simulink model "curr_vel_pos_cascaded"  (R2023b)
settings: Solver=VariableStepAuto  StartTime=0.0  StopTime=10  FixedStep=0.00001  RelTol=0.001
undefined symbols (not defined in the file or in its folder): d_theta, dd_theta, Fm, Im, theta
libraries: cstblocks x14
settings Model: Creator=frenci  LastModifiedBy=frenc

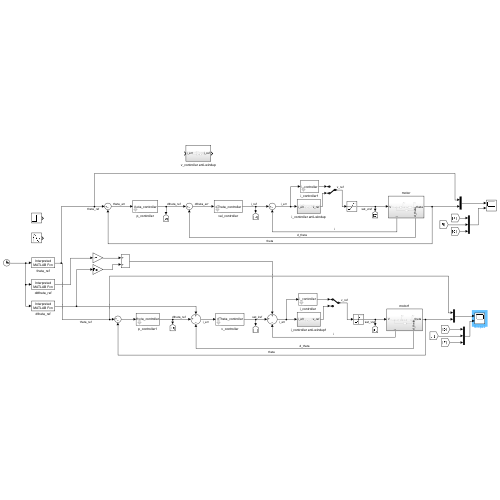
[thumbnail: Simulink's stored preview of the top-level diagram]
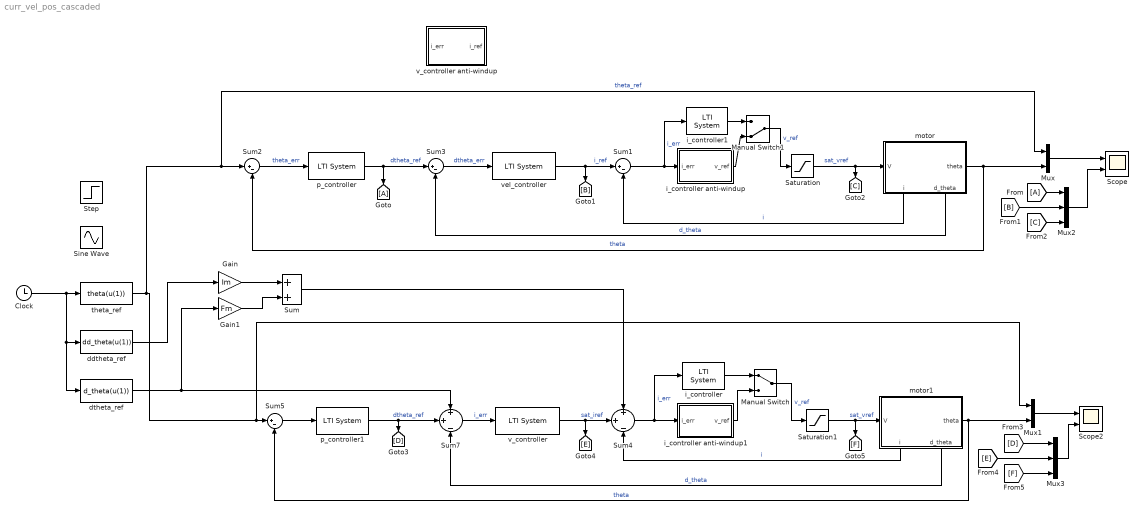
== system curr_vel_pos_cascaded ==
  Clock : Clock
  From : From
  Gain : Gain  Gain=Im
  Gain1 : Gain  Gain=Fm
  Goto : Goto
  Manual Switch : ManualSwitch
  Manual Switch1 : ManualSwitch  CurrentSetting=0
  Mux : Mux  Inputs=2
  Mux1 : Mux  Inputs=2
  Mux2 : Mux  Inputs=3
  Mux3 : Mux  Inputs=3
  Saturation : Saturate  UpperLimit=20  LowerLimit=-20
  Saturation1 : Saturate  UpperLimit=20  LowerLimit=-20
  Scope : Scope  NumInputPorts=2
  Scope2 : Scope  NumInputPorts=2
  Sine Wave : Sin  Amplitude=0.02  Frequency=2*pi*10  SampleTime=0
  Step : Step  Time=0.01  SampleTime=0
  Sum : Sum  Inputs=|+|+|
  Sum{1..3,5} (4 alike) : Sum  Inputs=|+-
  Sum4 : Sum  Inputs=+|+|-
  Sum7 : Sum  Inputs=+|+|-
  ddtheta_ref : MATLABFcn  MATLABFcn=dd_theta(u(1))
  dtheta_ref : MATLABFcn  MATLABFcn=d_theta(u(1))
  i_controller : cstblocks/LTI System  sys=i_controller  IC=[]  PadeOrder=0
  i_controller anti-windup : Subsystem
  i_controller anti-windup1 : Subsystem
  i_controller1 : cstblocks/LTI System  sys=i_controller  IC=[]  PadeOrder=0
  motor : Subsystem
      settings: PortSchema="{\"entries\":[{\"content\":{\"sides\":[{\"content\":{\"connectorIds\":[\"In1\"]},\"type\":\"ConnectorPlacement.EquallySpacedRectSide\",\"uuid\":\"f8a2075c-835e-4141-b12e-4d20e284e554\"},{\"content\":{\"connectorIds\":[\"Out1\"],\"side\":\"RIGHT\"},\"type\":\"ConnectorPlacement.EquallySpacedRectSide\",\"uuid\":\"7d0ccdb0-5eec-43bf-a9a0-3828bb795771\"},{\"content\":{\"side\":\"TOP\"},\"type\":\"ConnectorPlacement.EquallySpacedRectSide\",\"uuid\":\"6f2e9e0d-bcbc-45fe-ae47-d363e6343883\"},{\"content\":{\"connectorIds\":[\"Out2\",\"Out3\"],\"side\":\"BOTTOM\"},\"type\":\"ConnectorPlacement.EquallySpacedRectSide\",\"uuid\":\"12f63cf8-6157-4e53-9068-17bec2e9afdd\"}]},\"type\":\"ConnectorPlacement.EquallySpacedConnector\",\"uuid\":\"d79290fb-8e13-45e0-9c36-c4b7a16caadb\"}],\"packageUris\":[\"http://schema.mathworks.com/mf0/Connector/R2020b\"],\"version\":\"1.0\"}"
  motor1 : Subsystem
      settings: PortSchema="{\"entries\":[{\"content\":{\"sides\":[{\"content\":{\"connectorIds\":[\"In1\"]},\"type\":\"ConnectorPlacement.EquallySpacedRectSide\",\"uuid\":\"f8a2075c-835e-4141-b12e-4d20e284e554\"},{\"content\":{\"connectorIds\":[\"Out1\"],\"side\":\"RIGHT\"},\"type\":\"ConnectorPlacement.EquallySpacedRectSide\",\"uuid\":\"7d0ccdb0-5eec-43bf-a9a0-3828bb795771\"},{\"content\":{\"side\":\"TOP\"},\"type\":\"ConnectorPlacement.EquallySpacedRectSide\",\"uuid\":\"6f2e9e0d-bcbc-45fe-ae47-d363e6343883\"},{\"content\":{\"connectorIds\":[\"Out2\",\"Out3\"],\"side\":\"BOTTOM\"},\"type\":\"ConnectorPlacement.EquallySpacedRectSide\",\"uuid\":\"12f63cf8-6157-4e53-9068-17bec2e9afdd\"}]},\"type\":\"ConnectorPlacement.EquallySpacedConnector\",\"uuid\":\"d79290fb-8e13-45e0-9c36-c4b7a16caadb\"}],\"packageUris\":[\"http://schema.mathworks.com/mf0/Connector/R2020b\"],\"version\":\"1.0\"}"
  p_controller : cstblocks/LTI System  sys=theta_controller  IC=[]  PadeOrder=0
  p_controller1 : cstblocks/LTI System  sys=theta_controller  IC=[]  PadeOrder=0
  theta_ref : MATLABFcn  MATLABFcn=theta(u(1))
  v_controller : cstblocks/LTI System  sys=dTheta_controller  IC=[]  PadeOrder=0
  v_controller anti-windup : Subsystem
  vel_controller : cstblocks/LTI System  sys=dTheta_controller  IC=[]  PadeOrder=0
  wires:
  Sum2/1 -> p_controller/1  "theta_err"
  Mux/1 -> Scope/1
  motor/2(i) -> Sum1/2  "i"
  Saturation/1 -> [C], motor/1(V)  "sat_vref"
  vel_controller/1 -> Sum1/1, [B]  "i_ref"
  Sum1/1 -> i_controller1/1, i_controller anti-windup/1(i_err)  "i_err"
  i_controller anti-windup/1(v_ref) -> Manual Switch1/2
  Sum3/1 -> vel_controller/1  "dtheta_err"
  motor1/1(theta) -> Mux1/2, Sum5/2  "theta"
  Sum5/1 -> p_controller1/1
  motor1/2(i) -> Sum4/3  "i"
  Mux1/1 -> Scope2/1
  Saturation1/1 -> [F], motor1/1(V)  "sat_vref"
  p_controller1/1 -> Sum7/2, [D]  "dtheta_ref"
  v_controller/1 -> Sum4/2, [E]  "sat_iref"
  Clock/1 -> dtheta_ref/1, ddtheta_ref/1, theta_ref/1
  motor/3(d_theta) -> Sum3/2  "d_theta"
  theta_ref/1 -> Sum2/1, Mux/1, Sum5/1, Mux1/1  "theta_ref"
  p_controller/1 -> Sum3/1, Goto/1  "dtheta_ref"
  motor/1(theta) -> Mux/2, Sum2/2  "theta"
  Sum7/1 -> v_controller/1  "i_err"
  motor1/3(d_theta) -> Sum7/3  "d_theta"
  dtheta_ref/1 -> Gain1/1, Sum7/1
  [C] -> Mux2/3
  From/1 -> Mux2/1
  [B] -> Mux2/2
  Mux2/1 -> Scope/2
  [D] -> Mux3/1
  [F] -> Mux3/3
  [E] -> Mux3/2
  Mux3/1 -> Scope2/2
  i_controller/1 -> Manual Switch/1
  i_controller anti-windup1/1(v_ref) -> Manual Switch/2
  Manual Switch/1 -> Saturation1/1  "v_ref"
  Sum4/1 -> i_controller/1, i_controller anti-windup1/1(i_err)  "i_err"
  i_controller1/1 -> Manual Switch1/1
  Manual Switch1/1 -> Saturation/1  "v_ref"
  ddtheta_ref/1 -> Gain/1
  Gain/1 -> Sum/1
  Gain1/1 -> Sum/2
  Sum/1 -> Sum4/1

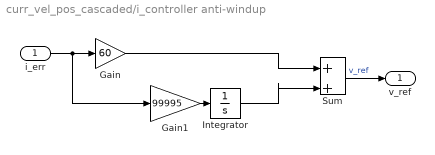
== system curr_vel_pos_cascaded/i_controller anti-windup ==
  i_err : Inport
  Gain : Gain  Gain=60
  Gain1 : Gain  Gain=99995
  Integrator : Integrator  LimitOutput=on  UpperSaturationLimit=5  LowerSaturationLimit=-5
  Sum : Sum  Inputs=|+||+|
  v_ref : Outport
  wires:
  i_err/1 -> Gain1/1, Gain/1
  Gain1/1 -> Integrator/1
  Gain/1 -> Sum/1
  Integrator/1 -> Sum/2
  Sum/1 -> v_ref/1  "v_ref"

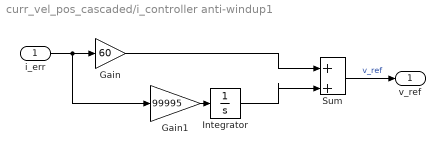
== system curr_vel_pos_cascaded/i_controller anti-windup1 ==
  i_err : Inport
  Gain : Gain  Gain=60
  Gain1 : Gain  Gain=99995
  Integrator : Integrator  LimitOutput=on  UpperSaturationLimit=5  LowerSaturationLimit=-5
  Sum : Sum  Inputs=|+||+|
  v_ref : Outport
  wires:
  i_err/1 -> Gain1/1, Gain/1
  Gain1/1 -> Integrator/1
  Gain/1 -> Sum/1
  Integrator/1 -> Sum/2
  Sum/1 -> v_ref/1  "v_ref"

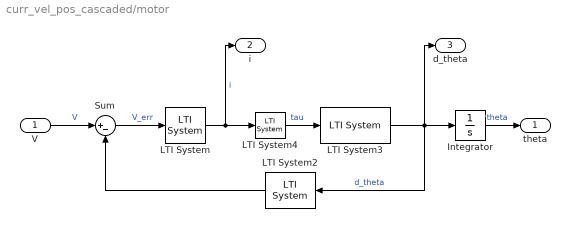
== system curr_vel_pos_cascaded/motor ==
  V : Inport
  Integrator : Integrator
  LTI System : cstblocks/LTI System  sys=El  IC=[]  PadeOrder=0
  LTI System2 : cstblocks/LTI System  sys=Kt  IC=[]  PadeOrder=0
  LTI System3 : cstblocks/LTI System  sys=Me  IC=[]  PadeOrder=0
  LTI System4 : cstblocks/LTI System  sys=Kt  IC=[]  PadeOrder=0
  Sum : Sum  Inputs=|+-
  theta : Outport
  i : Outport  Port=2
  d_theta : Outport  Port=3
  wires:
  LTI System2/1 -> Sum/2
  LTI System4/1 -> LTI System3/1  "tau"
  Integrator/1 -> theta/1  "theta"
  V/1 -> Sum/1  "V"
  Sum/1 -> LTI System/1  "V_err"
  LTI System3/1 -> d_theta/1, LTI System2/1, Integrator/1  "d_theta"
  LTI System/1 -> LTI System4/1, i/1  "i"

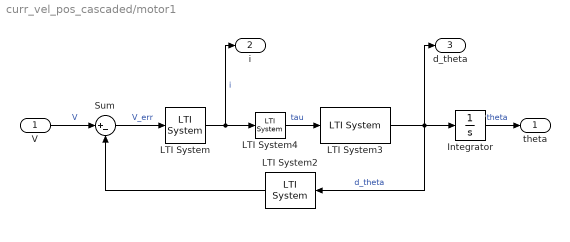
== system curr_vel_pos_cascaded/motor1 ==
  V : Inport
  Integrator : Integrator
  LTI System : cstblocks/LTI System  sys=El  IC=[]  PadeOrder=0
  LTI System2 : cstblocks/LTI System  sys=Kt  IC=[]  PadeOrder=0
  LTI System3 : cstblocks/LTI System  sys=Me  IC=[]  PadeOrder=0
  LTI System4 : cstblocks/LTI System  sys=Kt  IC=[]  PadeOrder=0
  Sum : Sum  Inputs=|+-
  theta : Outport
  i : Outport  Port=2
  d_theta : Outport  Port=3
  wires:
  LTI System2/1 -> Sum/2
  LTI System4/1 -> LTI System3/1  "tau"
  Integrator/1 -> theta/1  "theta"
  V/1 -> Sum/1  "V"
  Sum/1 -> LTI System/1  "V_err"
  LTI System3/1 -> d_theta/1, LTI System2/1, Integrator/1  "d_theta"
  LTI System/1 -> LTI System4/1, i/1  "i"

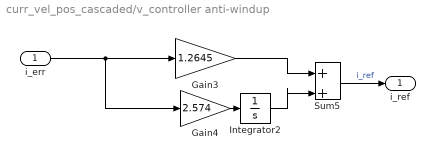
== system curr_vel_pos_cascaded/v_controller anti-windup ==
  i_err : Inport
  Gain3 : Gain  Gain=1.2645
  Gain4 : Gain  Gain=2.574
  Integrator2 : Integrator  LimitOutput=on  UpperSaturationLimit=1  LowerSaturationLimit=-1
  Sum5 : Sum  Inputs=|+||+|
  i_ref : Outport
  wires:
  Gain4/1 -> Integrator2/1
  Integrator2/1 -> Sum5/2
  Sum5/1 -> i_ref/1  "i_ref"
  Gain3/1 -> Sum5/1
  i_err/1 -> Gain4/1, Gain3/1
